simulink model "mealy__machine"  (R2020a)
settings: Solver=VariableStepAuto  StartTime=0.0  StopTime=10.0  RelTol=1e-3
settings Model: Creator=DELL  LastModifiedBy=DELL

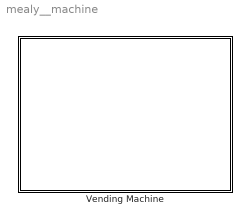
== system mealy__machine ==
  Vending Machine : Stateflow chart  TreatAsAtomicUnit=on

== stateflow chart mealy__machine/Vending Machine ==
  state Vending
  state Lime
  state Cola
  (default) -> Vending
  Vending -> Lime [order 1] : [coin == 1]{soda=0}
  Lime -> Vending [order 1] : [coin ==2]{soda=1}
  Cola -> Vending [order 1] : [coin==1]{soda=1}
  Vending -> Cola [order 2] : [coin==2]{soda=0}
  Lime -> Cola [order 2] : [coin==1]{soda=0}
  Cola -> Lime [order 2] : [coin==2]{soda=1}
